simulink library "ddm"  (R2021b)
settings: Solver=VariableStepAuto  StartTime=0.0  StopTime=10.0  RelTol=1e-3
undefined symbols (not defined in the file or in its folder): ADDM_FrTMTqDev_X_Nm, ADDM_RrTMTqDev_X_Nm, ENUM_ADASACCSTA_ERROR, ENUM_ADASACCSTA_OFF, ENUM_ADASACCSTA_STANDBY, ENUM_ALLOWMOV_ALLOWREADY, ENUM_APS, ENUM_BRKSTA_ERROR, ENUM_BRKSTA_OFF, ENUM_BRKSTA_ON, ENUM_BRKSW_INVALID, ENUM_BRKSW_OFF, ENUM_BRKSW_ON, ENUM_CHGPREACTERRSTA_OBCPRE, ENUM_DCDCFAULTSTA_ANYFAULTLV1, ENUM_DCDCFAULTSTA_ANYFAULTLV2, ENUM_DRIVETRAIN_AWD, ENUM_DRIVETRAIN_FWD, ENUM_DRIVETRAIN_RWD, ENUM_EDUDRTSTA_NORMAL, ENUM_EPBSTA_APPLIED, ENUM_EPBSTA_RELEASED, ENUM_GEARACTUALPOSN_INVALID, ENUM_GEARACTUALPOSN_P, ENUM_HVBATTREADYPRE_READY, ENUM_MCUWARN_LV0, ENUM_MCUWARN_LV1, ENUM_MCUWARN_LV2, ENUM_MCUWARN_LV3, ENUM_MCUWARN_NOERROR, ENUM_OBCFAULTSTA_ANYFAULT, ENUM_PAS_R2F2, ENUM_PDFAULT_BATTPDFAIL, ENUM_PDFAULT_DCDCDISABLE, ENUM_PDFAULT_MCUDISABLE, ENUM_PDFAULT_MCUDISCHRG, ENUM_POWERSTA_OFF, ENUM_POWERSTA_ON, ENUM_POWERSTA_READY, ENUM_POWERSTA_STANDBY, ENUM_PRESSINDI_LOW, ENUM_PUFAULT_BATTUPFAIL, ENUM_PUFAULT_DCDCENABLEFAIL, ENUM_PUFAULT_PRECHRGCHKFAIL, ENUM_PUFAULT_SAFETYCHKFAIL, ENUM_PUSTATE_COMPLETED, ENUM_PWRSTASW_OFF, ENUM_PWRSTASW_OFFA, ENUM_PWRSTASW_OFFCHVCHRG, ENUM_PWRSTASW_OFFCLVCHRG, ENUM_PWRSTASW_ON, ENUM_PWRSTASW_ONHVCHRG, ENUM_PWRSTASW_READY, ENUM_PWRSTASW_STANDBY, ENUM_SHIFTCOMMAND_P, ENUM_SHIFTERERRSTA_PBUTTONFAILURE, ENUM_VEHMALFUNLV_2ND, ENUM_VEHMALFUNLV_3RD, ENUM_VEHMALFUNLV_4TH, ENUM_VEHMALFUNLV_NORMAL ... (+459)
libraries: hcu_lib x515, simulink x3
(part 5 of 25)

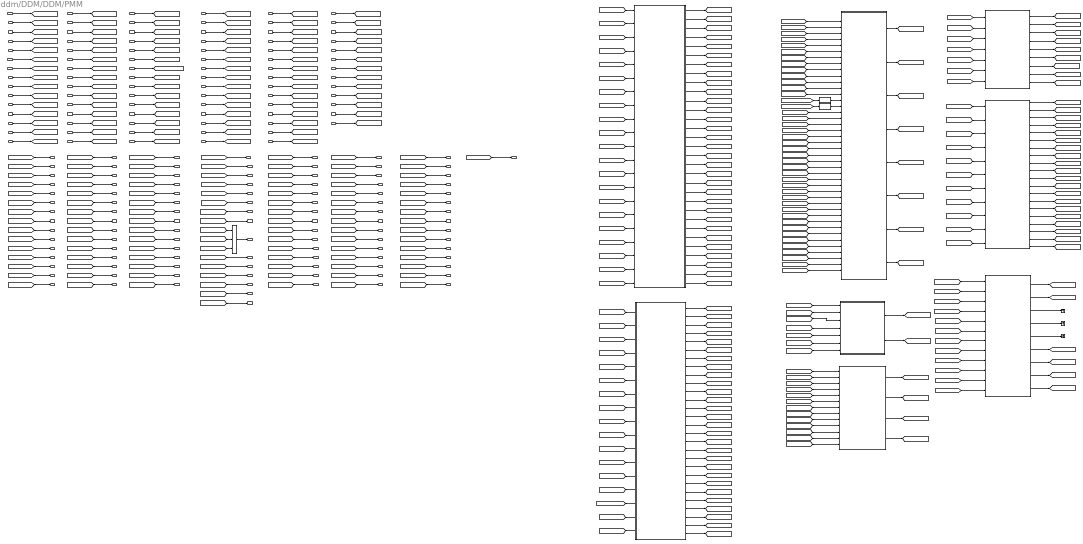
== system ddm/DDM/DDM/PMM ==
  task_time_s : Inport
  VINP_CANMsgValidABM1_flg : Inport  Port=2
  VINP_BrkPedalPosSta_enum : Inport  Port=3
  VINP_BrkPedalPos_pct : Inport  Port=4
  VINP_BrkSWSta_flg : Inport  Port=5
  VINP_CANMsgValidBMS1_flg : Inport  Port=6
  VINP_CANMsgValidBMS6_flg : Inport  Port=7
  VINP_CANMsgValidCCU1_flg : Inport  Port=8
  VINP_CANMsgValidCCU2_flg : Inport  Port=9
  VINP_BMSWarn1_flg : Inport  Port=10
  VINP_BMSWarn2_flg : Inport  Port=11
  VINP_BMSWarn3_flg : Inport  Port=12
  VINP_BMSWarn4_flg : Inport  Port=13
  VINP_BMSWarn5_flg : Inport  Port=14
  VINP_BMSWarn6_flg : Inport  Port=15
  VINP_BMSWarn7_flg : Inport  Port=16
  VINP_BMSWarn8_flg : Inport  Port=17
  VINP_DCDCFaultSta_enum : Inport  Port=18
  VINP_OBCFaultSta_enum : Inport  Port=19
  VINP_MCUWarnFNidec_enum : Inport  Port=20
  VINP_MCUWarnRNidec_enum : Inport  Port=21
  VINP_LVBattDet12V_V : Inport  Port=22
  VINP_BMSREADY_flg : Inport  Port=23
  VINP_HVBattReady4Pre_enum : Inport  Port=24
  VINP_HVBContactorSta_flg : Inport  Port=25
  VINP_DCDCReady4Pre_flg : Inport  Port=26
  VINP_DCDCEnabled_flg : Inport  Port=27
  VINP_CANMsgValidBMS5_flg : Inport  Port=28
  VINP_DrStdAErrSta_enum : Inport  Port=29
  VPMM_PowerSta_enum : Inport  Port=30
  VPMM_PwrStaSW_enum : Inport  Port=31
  VPMM_PowerUpFault_enum : Inport  Port=32
  VPMM_PowerDownFault_enum : Inport  Port=33
  VPMM_DrivetrainSelect_enum : Inport  Port=34
  VPMM_SafetyChkHLv_flg : Inport  Port=35
  VPMM_SafetyChkMLv_flg : Inport  Port=36
  VPMM_HVChrgPreActionErrSta_enum : Inport  Port=37
  VPMM_MCUReady_flg : Inport  Port=38
  VPMM_MCUReady4Pre_flg : Inport  Port=39
  VDDM_C3BMS6RCChk_flg : Inport  Port=40
  VDDM_C3BMS6CSChk_flg : Inport  Port=41
  VDDM_C3BMS1RCChk_flg : Inport  Port=42
  VDDM_C3BMS1CSChk_flg : Inport  Port=43
  VDDM_C3CCU1RCChk_flg : Inport  Port=44
  VDDM_C3CCU1CSChk_flg : Inport  Port=45
  VDDM_C3CCU2RCChk_flg : Inport  Port=46
  VDDM_C3CCU2CSChk_flg : Inport  Port=47
  VDDM_C1ABM1RCChk_flg : Inport  Port=48
  VDDM_C1ABM1CSChk_flg : Inport  Port=49
  VINP_BrakeSWGPIO_flg : Inport  Port=50
  VINP_BrakeLampSW_flg : Inport  Port=51
  VINP_DrStSW : Inport  Port=52
  VINP_FLAJARSW : Inport  Port=53
  VINP_FRAJARSW : Inport  Port=54
  VINP_RLAJARSW : Inport  Port=55
  VINP_RRAJARSW : Inport  Port=56
  VINP_HoodSW : Inport  Port=57
  VINP_TailgaSW : Inport  Port=58
  VDKC_DKCAuthSta_enum : Inport  Port=59
  VINP_AllowMovThd_OTA_enum : Inport  Port=60
  No_CAN1_BUS_OFF : Inport  Port=61
  No_CAN3_BUS_OFF : Inport  Port=62
  DTC_clear_request : Inport  Port=63
  VDDM_MCUNF1NoComCFS_flg : Inport  Port=64
  VDDM_MCUNR1NoComCFS_flg : Inport  Port=65
  VDDM_ESC5NoComCFS_flg : Inport  Port=66
  VDDM_ESC5RCErrCFS_flg : Inport  Port=67
  VDDM_ESC5CSErrCFS_flg : Inport  Port=68
  VPMM_PowerUpState_enum : Inport  Port=69
  VDDM_MCUNR1RCErrCFS_flg : Inport  Port=70
  VDDM_MCUNR1CSErrCFS_flg : Inport  Port=71
  VDDM_MCUNF1RCErrCFS_flg : Inport  Port=72
  VDDM_MCUNF1CSErrCFS_flg : Inport  Port=73
  VDDM_ESC1SigErr_flg : Inport  Port=74
  VDDM_ESC5SigErr_flg : Inport  Port=75
  VINP_ShifterFailsta_enum : Inport  Port=76
  VDDM_Shifter1NoComCFS_flg : Inport  Port=77
  VDDM_Shifter1RCErrCFS_flg : Inport  Port=78
  VDDM_Shifter1CSErrCFS_flg : Inport  Port=79
  No_CAN4_BUS_OFF : Inport  Port=80
  VINP_ZoneDrMalfunLevel_enum : Inport  Port=81
  VDDM_DrVCUNoComCFS_flg : Inport  Port=82
  ZoneFrMalfunLevel_enum : Inport  Port=83
  VDDM_FrVCUNoComCFS_flg : Inport  Port=84
  VDDM_AuxBattVolV_V : Inport  Port=85
  VPMM_MCUDCBusMaxVolt_V : Inport  Port=86
  VINP_CANMsgValidDKC1_flg : Inport  Port=87
  VINP_CANMsgValidDKC2_flg : Inport  Port=88
  Brake switch signal abnormal : Subsystem
  Comm err : Subsystem
  Data Type Conversion16 : DataTypeConversion  OutDataTypeStr=boolean
  Data Type Conversion49 : DataTypeConversion  OutDataTypeStr=boolean
  Fault level : Subsystem
  Key authentication failed : Subsystem
  LV : Subsystem
  Logical Operator5 : Logic  Operator=OR  Inputs=3  AllPortsSameDT=off  OutDataTypeStr=boolean
  SW failure : Subsystem
  System conditions of ON to READY not satisfied : Subsystem  AncestorBlock=ddm/DDM/DDM/PMM/System conditions of ON to READY not satisfied
  Terminator1 : Terminator
  Terminator10 : Terminator
  Terminator11 : Terminator
  power up and power down : Subsystem
  VDDM_C3BMS6RCDTC_raw32 : Outport
  VDDM_C3BMS6CSDTC_raw32 : Outport  Port=2
  VDDM_C3BMS6LCDTC_raw32 : Outport  Port=3
  VDDM_C3BMS1RCDTC_raw32 : Outport  Port=4
  VDDM_C3BMS1CSDTC_raw32 : Outport  Port=5
  VDDM_C3BMS1LCDTC_raw32 : Outport  Port=6
  VDDM_C3CCU1RCDTC_raw32 : Outport  Port=7
  VDDM_C3CCU1CSDTC_raw32 : Outport  Port=8
  VDDM_C3CCU1LCDTC_raw32 : Outport  Port=9
  VDDM_C3CCU2RCDTC_raw32 : Outport  Port=10
  VDDM_C3CCU2CSDTC_raw32 : Outport  Port=11
  VDDM_C3CCU2LCDTC_raw32 : Outport  Port=12
  VDDM_C1ABM1RCDTC_raw32 : Outport  Port=13
  VDDM_C1ABM1CSDTC_raw32 : Outport  Port=14
  VDDM_C1ABM1LCDTC_raw32 : Outport  Port=15
  VDDM_Lv1ErrDTC_raw32 : Outport  Port=16
  VDDM_Lv2ErrDTC_raw32 : Outport  Port=17
  VDDM_Lv3ErrDTC_raw32 : Outport  Port=18
  VDDM_Lv4ErrDTC_raw32 : Outport  Port=19
  VDDM_BrkSWErrDTC_raw32 : Outport  Port=20
  VDDM_BrkSWNoBacDTC_raw32 : Outport  Port=21
  VDDM_KeyAuthDTC_raw32 : Outport  Port=22
  VDDM_ONtoRdyDTC_raw32 : Outport  Port=23
  VDDM_HVB4PreDTC_raw32 : Outport  Port=24
  VDDM_MCU4PreDTC_raw32 : Outport  Port=25
  VDDM_DCDC4PreDTC_raw32 : Outport  Port=26
  VDDM_HVRlyCloDTC_raw32 : Outport  Port=27
  VDDM_BMSRdyDTC_raw32 : Outport  Port=28
  VDDM_DCDCEnaDTC_raw32 : Outport  Port=29
  VDDM_HiLvSaChkDTC_raw32 : Outport  Port=30
  VDDM_MidLvSaChkDTC_raw32 : Outport  Port=31
  VDDM_MCUDisDTC_raw32 : Outport  Port=32
  VDDM_DCDCDisDTC_raw32 : Outport  Port=33
  VDDM_HVRlyOpDTC_raw32 : Outport  Port=34
  VDDM_MCUActDTC_raw32 : Outport  Port=35
  VDDM_OBC4PreDTC_raw32 : Outport  Port=36
  VDDM_IniLVLoDTC_raw32 : Outport  Port=37
  VDDM_LVSupLoDTC_raw32 : Outport  Port=38
  VDDM_LVSupHiDTC_raw32 : Outport  Port=39
  VDDM_LVInErrDTC_raw32 : Outport  Port=40
  VDDM_DrStSWDTC_raw32 : Outport  Port=41
  VDDM_FLDoorSWDTC_raw32 : Outport  Port=42
  VDDM_RLDoorSWDTC_raw32 : Outport  Port=43
  VDDM_FRDoorSWDTC_raw32 : Outport  Port=44
  VDDM_RRDoorSWDTC_raw32 : Outport  Port=45
  VDDM_HoodSWDTC_raw32 : Outport  Port=46
  VDDM_TailgaSWDTC_raw32 : Outport  Port=47
  VDDM_VCUFLDoorSta_flg : Outport  Port=48
  VDDM_VCUFRDoorSta_flg : Outport  Port=49
  VDDM_VCURLDoorSta_flg : Outport  Port=50
  VDDM_VCURRDoorSta_flg : Outport  Port=51
  VDDM_VCUHoodSWSta_flg : Outport  Port=52
  VDDM_VCUTailgateSWSta_flg : Outport  Port=53
  VDDM_EDriveSysErrPMM_flg : Outport  Port=54
  VDDM_VCUBrkSWSta_enum : Outport  Port=55
  VDDM_SysAllowReadySta_flg : Outport  Port=56
  VDDM_HVRlyOpFail_flg : Outport  Port=57
  VDDM_MCUActDisFail_flg : Outport  Port=58
  VDDM_C3BMS6CSCFS_flg : Outport  Port=59
  VDDM_C3BMS6RCCFS_flg : Outport  Port=60
  VDDM_C3BMS6LCCFS_flg : Outport  Port=61
  VDDM_C3CCU2CSCFS_flg : Outport  Port=62
  VDDM_C3CCU2LCCFS_flg : Outport  Port=63
  VDDM_C3CCU2RCCFS_flg : Outport  Port=64
  VDDM_C3BMS1RCCFS_flg : Outport  Port=65
  VDDM_C3BMS1CSCFS_flg : Outport  Port=66
  VDDM_C3BMS1LCCFS_flg : Outport  Port=67
  VDDM_C3CCU1RCCFS_flg : Outport  Port=68
  VDDM_C3CCU1CSCFS_flg : Outport  Port=69
  VDDM_C3CCU1LCCFS_flg : Outport  Port=70
  VDDM_C1ABM1RCCFS_flg : Outport  Port=71
  VDDM_C1ABM1CSCFS_flg : Outport  Port=72
  VDDM_C1ABM1LCCFS_flg : Outport  Port=73
  VDDM_Lv1ErrCFS_flg : Outport  Port=74
  VDDM_Lv2ErrCFS_flg : Outport  Port=75
  VDDM_Lv3ErrCFS_flg : Outport  Port=76
  VDDM_Lv4ErrCFS_flg : Outport  Port=77
  VDDM_IniLVLoCFS_flg : Outport  Port=78
  VDDM_LVSupLoCFS_flg : Outport  Port=79
  VDDM_LVSupHiCFS_flg : Outport  Port=80
  VDDM_LVInErrCFS_flg : Outport  Port=81
  VDDM_HVB4PreCFS_flg : Outport  Port=82
  VDDM_MCU4PreCFS_flg : Outport  Port=83
  VDDM_DCDC4PreCFS_flg : Outport  Port=84
  VDDM_HVRlyCloCFS_flg : Outport  Port=85
  VDDM_BMSRdyCFS_flg : Outport  Port=86
  VDDM_DCDCEnaCFS_flg : Outport  Port=87
  VDDM_HiLvSaChkCFS_flg : Outport  Port=88
  VDDM_MidLvSaChkCFS_flg : Outport  Port=89
  VDDM_MCUDisCFS_flg : Outport  Port=90
  VDDM_DCDCDisCFS_flg : Outport  Port=91
  VDDM_HVRlyOpCFS_flg : Outport  Port=92
  VDDM_MCUActCFS_flg : Outport  Port=93
  VDDM_OBC4PreCFS_flg : Outport  Port=94
  VDDM_KeyAuthCFS_flg : Outport  Port=95
  VDDM_ONtoRdyCFS_flg : Outport  Port=96
  VDDM_DrStSWCFS_flg : Outport  Port=97
  VDDM_FLDoorSWCFS_flg : Outport  Port=98
  VDDM_RLDoorSWCFS_flg : Outport  Port=99
  VDDM_FRDoorSWCFS_flg : Outport  Port=100
  VDDM_RRDoorSWCFS_flg : Outport  Port=101
  VDDM_HoodSWCFS_flg : Outport  Port=102
  VDDM_TailgaSWCFS_flg : Outport  Port=103
  VDDM_BrkSWErrCFS_flg : Outport  Port=104
  VDDM_BrkSWNoBacCFS_flg : Outport  Port=105
  VDDM_PMMBattErr_flg : Outport  Port=106
  wires:
  [VDDM_SysAllowReadySta_flg] -> VDDM_SysAllowReadySta_flg/1
  [VDDM_VCUBrkSWSta_enum] -> VDDM_VCUBrkSWSta_enum/1
  [VDDM_C3CCU2RCCFS_flg] -> VDDM_C3CCU2RCCFS_flg/1
  [VDDM_C3CCU2LCCFS_flg] -> VDDM_C3CCU2LCCFS_flg/1
  [VDDM_C3CCU2CSCFS_flg] -> VDDM_C3CCU2CSCFS_flg/1
  [VDDM_C3BMS6LCCFS_flg] -> VDDM_C3BMS6LCCFS_flg/1
  [VDDM_C3BMS6RCCFS_flg] -> VDDM_C3BMS6RCCFS_flg/1
  [VDDM_C3BMS6CSCFS_flg] -> VDDM_C3BMS6CSCFS_flg/1
  Comm err/17(VDDM_C3BMS6CSCFS_flg) -> [VDDM_C3BMS6CSCFS_flg]
  [VPMM_PowerUpState_enum] -> power up and power down/16(VPMM_PowerUpState_enum)
  VPMM_PowerUpState_enum/1 -> [VPMM_PowerUpState_enum]
  Data Type Conversion16/1 -> Fault level/15(VDDM_C3CCU2LCCFS_flg)
  [VDDM_C3CCU2LCDTC_raw32] -> Data Type Conversion16/1
  Data Type Conversion49/1 -> Fault level/14(VDDM_C3BMS6LCCFS_flg)
  [No_CAN3_BUS_OFF] -> Fault level/22(No_CAN3_BUS_OFF)
  [DTC_clear_request] -> Fault level/21(DTC_clear_request)
  [VDDM_C3BMS6LCDTC_raw32] -> Data Type Conversion49/1
  VDDM_ESC5CSErrCFS_flg/1 -> [VDDM_ESC5CSErrCFS_flg]
  VDDM_ESC5RCErrCFS_flg/1 -> [VDDM_ESC5RCErrCFS_flg]
  VDDM_ESC5NoComCFS_flg/1 -> [VDDM_ESC5NoComCFS_flg]
  VDDM_MCUNR1NoComCFS_flg/1 -> [VDDM_MCUNR1NoComCFS_flg]
  VDDM_MCUNF1NoComCFS_flg/1 -> [VDDM_MCUNF1NoComCFS_flg]
  [VDDM_KeyAuthDTC_raw32] -> VDDM_KeyAuthDTC_raw32/1
  Brake switch signal abnormal/5(VDDM_BrkPedalPosSta_enum) -> Terminator11/1
  Brake switch signal abnormal/4(VDDM_CANBrkSW2Sta_enum) -> Terminator10/1
  System conditions of ON to READY not satisfied/4(VDDM_SysAllowReadySta_flg) -> [VDDM_SysAllowReadySta_flg]
  [VDDM_C3BMS6CSDTC_raw32] -> VDDM_C3BMS6CSDTC_raw32/1
  [VDDM_C3BMS6LCDTC_raw32] -> VDDM_C3BMS6LCDTC_raw32/1
  [VDDM_C3BMS1RCDTC_raw32] -> VDDM_C3BMS1RCDTC_raw32/1
  [VDDM_C3BMS6RCDTC_raw32] -> VDDM_C3BMS6RCDTC_raw32/1
  [VDDM_C1ABM1LCDTC_raw32] -> VDDM_C1ABM1LCDTC_raw32/1
  [VDDM_C1ABM1CSDTC_raw32] -> VDDM_C1ABM1CSDTC_raw32/1
  [VDDM_C1ABM1RCDTC_raw32] -> VDDM_C1ABM1RCDTC_raw32/1
  [VDDM_C3CCU2LCDTC_raw32] -> VDDM_C3CCU2LCDTC_raw32/1
  [VDDM_C3CCU2CSDTC_raw32] -> VDDM_C3CCU2CSDTC_raw32/1
  [VDDM_C3CCU2RCDTC_raw32] -> VDDM_C3CCU2RCDTC_raw32/1
  [VDDM_C3CCU1LCDTC_raw32] -> VDDM_C3CCU1LCDTC_raw32/1
  [VDDM_C3CCU1CSDTC_raw32] -> VDDM_C3CCU1CSDTC_raw32/1
  [VDDM_C3CCU1RCDTC_raw32] -> VDDM_C3CCU1RCDTC_raw32/1
  [VDDM_C3BMS1LCDTC_raw32] -> VDDM_C3BMS1LCDTC_raw32/1
  [VDDM_C3BMS1CSDTC_raw32] -> VDDM_C3BMS1CSDTC_raw32/1
  Comm err/15(VDDM_C1ABM1LCDTC_raw32) -> [VDDM_C1ABM1LCDTC_raw32]
  Comm err/14(VDDM_C1ABM1CSDTC_raw32) -> [VDDM_C1ABM1CSDTC_raw32]
  Comm err/13(VDDM_C1ABM1RCDTC_raw32) -> [VDDM_C1ABM1RCDTC_raw32]
  Comm err/12(VDDM_C3CCU2LCDTC_raw32) -> [VDDM_C3CCU2LCDTC_raw32]
  Comm err/11(VDDM_C3CCU2CSDTC_raw32) -> [VDDM_C3CCU2CSDTC_raw32]
  Comm err/10(VDDM_C3CCU2RCDTC_raw32) -> [VDDM_C3CCU2RCDTC_raw32]
  Comm err/9(VDDM_C3CCU1LCDTC_raw32) -> [VDDM_C3CCU1LCDTC_raw32]
  Comm err/8(VDDM_C3CCU1CSDTC_raw32) -> [VDDM_C3CCU1CSDTC_raw32]
  Comm err/7(VDDM_C3CCU1RCDTC_raw32) -> [VDDM_C3CCU1RCDTC_raw32]
  Comm err/6(VDDM_C3BMS1LCDTC_raw32) -> [VDDM_C3BMS1LCDTC_raw32]
  Comm err/5(VDDM_C3BMS1CSDTC_raw32) -> [VDDM_C3BMS1CSDTC_raw32]
  Comm err/4(VDDM_C3BMS1RCDTC_raw32) -> [VDDM_C3BMS1RCDTC_raw32]
  Comm err/3(VDDM_C3BMS6LCDTC_raw32) -> [VDDM_C3BMS6LCDTC_raw32]
  Comm err/2(VDDM_C3BMS6CSDTC_raw32) -> [VDDM_C3BMS6CSDTC_raw32]
  Comm err/1(VDDM_C3BMS6RCDTC_raw32) -> [VDDM_C3BMS6RCDTC_raw32]
  [VPMM_PwrStaSW_enum] -> Key authentication failed/3(VPMM_PwrStaSW_enum)
  [VPMM_PowerSta_enum] -> System conditions of ON to READY not satisfied/2(VPMM_PowerSta_enum)
  System conditions of ON to READY not satisfied/3(VDDM_EDriveSysErrONtoRdy_flg) -> [VDDM_EDriveSysErrONtoRdy_flg]
  [DTC_clear_request] -> Brake switch signal abnormal/12(DTC_clear_request)
  [VINP_LVBattDet12V_V] -> LV/4(VINP_LVBattDet12V_V)
  No_CAN3_BUS_OFF/1 -> [No_CAN3_BUS_OFF]
  VDDM_C3BMS1CSChk_flg/1 -> [VDDM_C3BMS1CSChk_flg]
  [VDDM_EDriveSysErrBrake_flg] -> Logical Operator5/3
  [DTC_clear_request] -> LV/6(DTC_clear_request)
  [VDDM_MCUNF1NoComCFS_flg] -> Fault level/16(VDDM_MCUNF1NoComCFS_flg)
  DTC_clear_request/1 -> [DTC_clear_request]
  [VDDM_ESC5RCErrCFS_flg] -> Brake switch signal abnormal/6(VDDM_ESC5RCErrCFS_flg)
  [VDDM_EDriveSysErrONtoRdy_flg] -> Logical Operator5/2
  [VDDM_KeyAuthCFS_flg] -> System conditions of ON to READY not satisfied/7(VDDM_KeyAuthCFS_flg)
  [VDDM_MCUNR1NoComCFS_flg] -> Fault level/17(VDDM_MCUNR1NoComCFS_flg)
  [VPMM_PowerSta_enum] -> Comm err/2(VPMM_PowerSta_enum)
  [VPMM_PowerSta_enum] -> LV/3(VPMM_PowerSta_enum)
  [DTC_clear_request] -> SW failure/4(DTC_clear_request)
  [VDDM_C3CCU1RCChk_flg] -> Comm err/10(VDDM_C3CCU1RCChk_flg)
  [DTC_clear_request] -> System conditions of ON to READY not satisfied/4(DTC_clear_request)
  [VDDM_C1ABM1RCChk_flg] -> Comm err/16(VDDM_C1ABM1RCChk_flg)
  VPMM_PowerSta_enum/1 -> [VPMM_PowerSta_enum]
  [VDDM_ESC5CSErrCFS_flg] -> Brake switch signal abnormal/7(VDDM_ESC5CSErrCFS_flg)
  [task_time_s] -> System conditions of ON to READY not satisfied/1(task_time_s)
  Logical Operator5/1 -> VDDM_EDriveSysErrPMM_flg/1
  VINP_CANMsgValidABM1_flg/1 -> [VDDM_C1ABM1LCChk_flg]
  [VINP_CANMsgValidBMS5_flg] -> LV/5(VINP_CANMsgValidBMS5_flg)
  [VDDM_C3CCU2LCChk_flg] -> Comm err/15(VDDM_C3CCU2LCChk_flg)
  [VDDM_C1ABM1CSChk_flg] -> Comm err/17(VDDM_C1ABM1CSChk_flg)
  VDDM_C1ABM1RCChk_flg/1 -> [VDDM_C1ABM1RCChk_flg]
  [No_CAN1_BUS_OFF] -> Comm err/20(No_CAN1_BUS_OFF)
  [VDDM_EDriveSysErrABMCAN_flg] -> Logical Operator5/1
  VDDM_C3BMS1RCChk_flg/1 -> [VDDM_C3BMS1RCChk_flg]
  [VDDM_C3CCU1LCChk_flg] -> Comm err/12(VDDM_C3CCU1LCChk_flg)
  VPMM_PwrStaSW_enum/1 -> [VPMM_PwrStaSW_enum]
  [VPMM_PowerSta_enum] -> Key authentication failed/2(VPMM_PowerSta_enum)
  [VPMM_PwrStaSW_enum] -> System conditions of ON to READY not satisfied/3(VPMM_PwrStaSW_enum)
  [VPMM_PwrStaSW_enum] -> Comm err/3(VPMM_PwrStaSW_enum)
  [DTC_clear_request] -> power up and power down/6(DTC_clear_request)
  [VDDM_C1ABM1LCChk_flg] -> Comm err/18(VDDM_C1ABM1LCChk_flg)
  VDDM_C3CCU2RCChk_flg/1 -> [VDDM_C3CCU2RCChk_flg]
  [task_time_s] -> power up and power down/1(task_time_s)
  [task_time_s] -> LV/1(task_time_s)
  [VDDM_C3CCU1CSChk_flg] -> Comm err/11(VDDM_C3CCU1CSChk_flg)
  [VPMM_PowerSta_enum] -> power up and power down/3(VPMM_PowerSta_enum)
  VDDM_C1ABM1CSChk_flg/1 -> [VDDM_C1ABM1CSChk_flg]
  [VDDM_C3BMS1RCChk_flg] -> Comm err/7(VDDM_C3BMS1RCChk_flg)
  VINP_CANMsgValidCCU2_flg/1 -> [VDDM_C3CCU2LCChk_flg]
  [VPMM_PwrStaSW_enum] -> LV/2(VPMM_PwrStaSW_enum)
  Brake switch signal abnormal/3(VDDM_BrakeSW_enum) -> Terminator1/1
  VINP_LVBattDet12V_V/1 -> [VINP_LVBattDet12V_V]
  [task_time_s] -> Comm err/1(task_time_s)
  Comm err/31(VDDM_EDriveSysErrABMCAN_flg) -> [VDDM_EDriveSysErrABMCAN_flg]
  [VDDM_C3CCU2CSChk_flg] -> Comm err/14(VDDM_C3CCU2CSChk_flg)
  VINP_BrakeLampSW_flg/1 -> [VINP_BrakeLampSW_flg]
  [VPMM_PowerSta_enum] -> Brake switch signal abnormal/2(VPMM_PowerSta_enum)
  VDDM_C3CCU1RCChk_flg/1 -> [VDDM_C3CCU1RCChk_flg]
  [task_time_s] -> Fault level/1(task_time_s)
  [VPMM_PowerSta_enum] -> Fault level/3(VPMM_PowerSta_enum)
  [VDDM_C3BMS6CSChk_flg] -> Comm err/5(VDDM_C3BMS6CSChk_flg)
  [VINP_BrakeLampSW_flg] -> Brake switch signal abnormal/4(VINP_BrakeLampSW_flg)
  VDDM_C3BMS6CSChk_flg/1 -> [VDDM_C3BMS6CSChk_flg]
  VINP_BrakeSWGPIO_flg/1 -> [VINP_BrakeSWGPIO_flg]
  [VPMM_PwrStaSW_enum] -> SW failure/2(VPMM_PwrStaSW_enum)
  [VDDM_C3BMS6RCChk_flg] -> Comm err/4(VDDM_C3BMS6RCChk_flg)
  [VDDM_ESC5NoComCFS_flg] -> Brake switch signal abnormal/5(VDDM_ESC5NoComCFS_flg)
  [No_CAN3_BUS_OFF] -> Comm err/19(No_CAN3_BUS_OFF)
  [task_time_s] -> SW failure/1(task_time_s)
  [VPMM_PwrStaSW_enum] -> power up and power down/2(VPMM_PwrStaSW_enum)
  [task_time_s] -> Brake switch signal abnormal/1(task_time_s)
  [DTC_clear_request] -> Comm err/21(DTC_clear_request)
  [VPMM_PowerSta_enum] -> SW failure/3(VPMM_PowerSta_enum)
  VDDM_C3BMS6RCChk_flg/1 -> [VDDM_C3BMS6RCChk_flg]
  VINP_CANMsgValidBMS6_flg/1 -> [VDDM_C3BMS6LCChk_flg]
  [DTC_clear_request] -> Key authentication failed/4(DTC_clear_request)
  [task_time_s] -> Key authentication failed/1(task_time_s)
  VDDM_C3CCU1CSChk_flg/1 -> [VDDM_C3CCU1CSChk_flg]
  VDDM_C3CCU2CSChk_flg/1 -> [VDDM_C3CCU2CSChk_flg]
  [VPMM_PwrStaSW_enum] -> Fault level/2(VPMM_PwrStaSW_enum)
  [VDDM_C3CCU2RCChk_flg] -> Comm err/13(VDDM_C3CCU2RCChk_flg)
  [VINP_BrakeSWGPIO_flg] -> Brake switch signal abnormal/3(VINP_BrakeSWGPIO_flg)
  [VDDM_C3BMS1LCChk_flg] -> Comm err/9(VDDM_C3BMS1LCChk_flg)
  task_time_s/1 -> [task_time_s]
  No_CAN1_BUS_OFF/1 -> [No_CAN1_BUS_OFF]
  [VDDM_C3BMS1CSChk_flg] -> Comm err/8(VDDM_C3BMS1CSChk_flg)
  VINP_CANMsgValidCCU1_flg/1 -> [VDDM_C3CCU1LCChk_flg]
  [VDDM_C3BMS6LCChk_flg] -> Comm err/6(VDDM_C3BMS6LCChk_flg)
  Comm err/16(VDDM_C3BMS6RCCFS_flg) -> [VDDM_C3BMS6RCCFS_flg]
  Comm err/18(VDDM_C3BMS6LCCFS_flg) -> [VDDM_C3BMS6LCCFS_flg]
  Comm err/19(VDDM_C3BMS1RCCFS_flg) -> [VDDM_C3BMS1RCCFS_flg]
  Comm err/20(VDDM_C3BMS1CSCFS_flg) -> [VDDM_C3BMS1CSCFS_flg]
  Comm err/21(VDDM_C3BMS1LCCFS_flg) -> [VDDM_C3BMS1LCCFS_flg]
  Comm err/22(VDDM_C3CCU1RCCFS_flg) -> [VDDM_C3CCU1RCCFS_flg]
  Comm err/23(VDDM_C3CCU1CSCFS_flg) -> [VDDM_C3CCU1CSCFS_flg]
  Comm err/24(VDDM_C3CCU1LCCFS_flg) -> [VDDM_C3CCU1LCCFS_flg]
  Comm err/25(VDDM_C3CCU2RCCFS_flg) -> [VDDM_C3CCU2RCCFS_flg]
  Comm err/26(VDDM_C3CCU2CSCFS_flg) -> [VDDM_C3CCU2CSCFS_flg]
  Comm err/27(VDDM_C3CCU2LCCFS_flg) -> [VDDM_C3CCU2LCCFS_flg]
  Comm err/28(VDDM_C1ABM1RCCFS_flg) -> [VDDM_C1ABM1RCCFS_flg]
  Comm err/29(VDDM_C1ABM1CSCFS_flg) -> [VDDM_C1ABM1CSCFS_flg]
  Comm err/30(VDDM_C1ABM1LCCFS_flg) -> [VDDM_C1ABM1LCCFS_flg]
  power up and power down/16(VDDM_HVB4PreCFS_flg) -> [VDDM_HVB4PreCFS_flg]
  power up and power down/17(VDDM_MCU4PreCFS_flg) -> [VDDM_MCU4PreCFS_flg]
  power up and power down/18(VDDM_DCDC4PreCFS_flg) -> [VDDM_DCDC4PreCFS_flg]
  power up and power down/19(VDDM_HVRlyCloCFS_flg) -> [VDDM_HVRlyCloCFS_flg]
  power up and power down/20(VDDM_BMSRdyCFS_flg) -> [VDDM_BMSRdyCFS_flg]
  power up and power down/21(VDDM_DCDCEnaCFS_flg) -> [VDDM_DCDCEnaCFS_flg]
  power up and power down/22(VDDM_HiLvSaChkCFS_flg) -> [VDDM_HiLvSaChkCFS_flg]
  power up and power down/23(VDDM_MidLvSaChkCFS_flg) -> [VDDM_MidLvSaChkCFS_flg]
  power up and power down/24(VDDM_MCUDisCFS_flg) -> [VDDM_MCUDisCFS_flg]
  power up and power down/25(VDDM_DCDCDisCFS_flg) -> [VDDM_DCDCDisCFS_flg]
  power up and power down/26(VDDM_HVRlyOpCFS_flg) -> [VDDM_HVRlyOpCFS_flg]
  power up and power down/27(VDDM_MCUActCFS_flg) -> [VDDM_MCUActCFS_flg]
  power up and power down/28(VDDM_OBC4PreCFS_flg) -> [VDDM_OBC4PreCFS_flg]
  Fault level/5(VDDM_Lv1ErrCFS_flg) -> [VDDM_Lv1ErrCFS_flg]
  Fault level/6(VDDM_Lv2ErrCFS_flg) -> [VDDM_Lv2ErrCFS_flg]
  Fault level/7(VDDM_Lv3ErrCFS_flg) -> [VDDM_Lv3ErrCFS_flg]
  Fault level/8(VDDM_Lv4ErrCFS_flg) -> [VDDM_Lv4ErrCFS_flg]
  LV/5(VDDM_IniLVLoCFS_flg) -> [VDDM_IniLVLoCFS_flg]
  LV/6(VDDM_LVSupLoCFS_flg) -> [VDDM_LVSupLoCFS_flg]
  LV/7(VDDM_LVSupHiCFS_flg) -> [VDDM_LVSupHiCFS_flg]
  LV/8(VDDM_LVInErrCFS_flg) -> [VDDM_LVInErrCFS_flg]
  SW failure/14(VDDM_DrStSWCFS_flg) -> [VDDM_DrStSWCFS_flg]
  SW failure/15(VDDM_FLDoorSWCFS_flg) -> [VDDM_FLDoorSWCFS_flg]
  SW failure/16(VDDM_RLDoorSWCFS_flg) -> [VDDM_RLDoorSWCFS_flg]
  SW failure/17(VDDM_FRDoorSWCFS_flg) -> [VDDM_FRDoorSWCFS_flg]
  SW failure/18(VDDM_RRDoorSWCFS_flg) -> [VDDM_RRDoorSWCFS_flg]
  SW failure/19(VDDM_HoodSWCFS_flg) -> [VDDM_HoodSWCFS_flg]
  SW failure/20(VDDM_TailgaSWCFS_flg) -> [VDDM_TailgaSWCFS_flg]
  [VDDM_C3CCU2RCCFS_flg] -> Fault level/23(VDDM_C3CCU2RCCFS_flg)
  [VDDM_C3CCU2CSCFS_flg] -> Fault level/24(VDDM_C3CCU2CSCFS_flg)
  [VDDM_MCUNR1RCErrCFS_flg] -> Fault level/25(VDDM_MCUNR1RCErrCFS_flg)
  [VDDM_MCUNR1CSErrCFS_flg] -> Fault level/26(VDDM_MCUNR1CSErrCFS_flg)
  [VDDM_MCUNF1RCErrCFS_flg] -> Fault level/27(VDDM_MCUNF1RCErrCFS_flg)
  [VDDM_MCUNF1CSErrCFS_flg] -> Fault level/28(VDDM_MCUNF1CSErrCFS_flg)
  [VDDM_C3BMS6RCCFS_flg] -> Fault level/29(VDDM_C3BMS6RCCFS_flg)
  [VDDM_C3BMS6CSCFS_flg] -> Fault level/30(VDDM_C3BMS6CSCFS_flg)
  [VDDM_ESC1SigErr_flg] -> Fault level/32(VDDM_ESC1SigErr_flg)
  [VDDM_ESC5SigErr_flg] -> Fault level/33(VDDM_ESC5SigErr_flg)
  [No_CAN1_BUS_OFF] -> Fault level/31(No_CAN1_BUS_OFF)
  [ZoneFrMalfunLevel_enum] -> Fault level/34(ZoneFrMalfunLevel_enum)
  [VDDM_FrVCUNoComCFS_flg] -> Fault level/35(VDDM_FrVCUNoComCFS_flg)
  [VINP_ShifterFailsta_enum] -> Fault level/36(VINP_ShifterFailsta_enum)
  [VDDM_Shifter1NoComCFS_flg] -> Fault level/37(VDDM_Shifter1NoComCFS_flg)
  [VDDM_Shifter1RCErrCFS_flg] -> Fault level/38(VDDM_Shifter1RCErrCFS_flg)
  [VDDM_Shifter1CSErrCFS_flg] -> Fault level/39(VDDM_Shifter1CSErrCFS_flg)
  [VINP_ZoneDrMalfunLevel_enum] -> Fault level/40(VINP_ZoneDrMalfunLevel_enum)
  [No_CAN4_BUS_OFF] -> Fault level/41(No_CAN4_BUS_OFF)
  [VDDM_DrVCUNoComCFS_flg] -> Fault level/42(VDDM_DrVCUNoComCFS_flg)
  Brake switch signal abnormal/8(VDDM_VCUBrkSWSta_enum) -> [VDDM_VCUBrkSWSta_enum]
  Brake switch signal abnormal/9(VDDM_EDriveSysErrBrake_flg) -> [VDDM_EDriveSysErrBrake_flg]
  Brake switch signal abnormal/6(VDDM_BrkSWErrCFS_flg) -> [VDDM_BrkSWErrCFS_flg]
  Brake switch signal abnormal/7(VDDM_BrkSWNoBacCFS_flg) -> [VDDM_BrkSWNoBacCFS_flg]
  Key authentication failed/1(VDDM_KeyAuthDTC_raw32) -> [VDDM_KeyAuthDTC_raw32]
  Key authentication failed/2(VDDM_KeyAuthCFS_flg) -> [VDDM_KeyAuthCFS_flg]
  [VDDM_FLDoorSWCFS_flg] -> System conditions of ON to READY not satisfied/8(VDDM_FLDoorSWCFS_flg)
  [VDDM_RLDoorSWCFS_flg] -> System conditions of ON to READY not satisfied/9(VDDM_RLDoorSWCFS_flg)
  [VDDM_RRDoorSWCFS_flg] -> System conditions of ON to READY not satisfied/11(VDDM_RRDoorSWCFS_flg)
  [VDDM_FRDoorSWCFS_flg] -> System conditions of ON to READY not satisfied/10(VDDM_FRDoorSWCFS_flg)
  [VDDM_HoodSWCFS_flg] -> System conditions of ON to READY not satisfied/12(VDDM_HoodSWCFS_flg)
  [VDDM_TailgaSWCFS_flg] -> System conditions of ON to READY not satisfied/13(VDDM_TailgaSWCFS_flg)
  System conditions of ON to READY not satisfied/2(VDDM_ONtoRdyCFS_flg) -> [VDDM_ONtoRdyCFS_flg]
  [VDDM_C3BMS1RCCFS_flg] -> VDDM_C3BMS1RCCFS_flg/1
  [VDDM_C3BMS1CSCFS_flg] -> VDDM_C3BMS1CSCFS_flg/1
  [VDDM_C3BMS1LCCFS_flg] -> VDDM_C3BMS1LCCFS_flg/1
  [VDDM_C3CCU1RCCFS_flg] -> VDDM_C3CCU1RCCFS_flg/1
  [VDDM_C3CCU1CSCFS_flg] -> VDDM_C3CCU1CSCFS_flg/1
  [VDDM_C3CCU1LCCFS_flg] -> VDDM_C3CCU1LCCFS_flg/1
  [VDDM_C1ABM1RCCFS_flg] -> VDDM_C1ABM1RCCFS_flg/1
  [VDDM_C1ABM1CSCFS_flg] -> VDDM_C1ABM1CSCFS_flg/1
  [VDDM_C1ABM1LCCFS_flg] -> VDDM_C1ABM1LCCFS_flg/1
  [VDDM_Lv1ErrCFS_flg] -> VDDM_Lv1ErrCFS_flg/1
  [VDDM_Lv2ErrCFS_flg] -> VDDM_Lv2ErrCFS_flg/1
  [VDDM_Lv3ErrCFS_flg] -> VDDM_Lv3ErrCFS_flg/1
  [VDDM_Lv4ErrCFS_flg] -> VDDM_Lv4ErrCFS_flg/1
  [VDDM_IniLVLoCFS_flg] -> VDDM_IniLVLoCFS_flg/1
  [VDDM_LVSupLoCFS_flg] -> VDDM_LVSupLoCFS_flg/1
  [VDDM_LVSupHiCFS_flg] -> VDDM_LVSupHiCFS_flg/1
  [VDDM_LVInErrCFS_flg] -> VDDM_LVInErrCFS_flg/1
  [VDDM_HVB4PreCFS_flg] -> VDDM_HVB4PreCFS_flg/1
  [VDDM_MCU4PreCFS_flg] -> VDDM_MCU4PreCFS_flg/1
  [VDDM_DCDC4PreCFS_flg] -> VDDM_DCDC4PreCFS_flg/1
  [VDDM_HVRlyCloCFS_flg] -> VDDM_HVRlyCloCFS_flg/1
  [VDDM_BMSRdyCFS_flg] -> VDDM_BMSRdyCFS_flg/1
  [VDDM_DCDCEnaCFS_flg] -> VDDM_DCDCEnaCFS_flg/1
  [VDDM_HiLvSaChkCFS_flg] -> VDDM_HiLvSaChkCFS_flg/1
  [VDDM_MidLvSaChkCFS_flg] -> VDDM_MidLvSaChkCFS_flg/1
  [VDDM_MCUDisCFS_flg] -> VDDM_MCUDisCFS_flg/1
  [VDDM_DCDCDisCFS_flg] -> VDDM_DCDCDisCFS_flg/1
  [VDDM_HVRlyOpCFS_flg] -> VDDM_HVRlyOpCFS_flg/1
  [VDDM_MCUActCFS_flg] -> VDDM_MCUActCFS_flg/1
  [VDDM_OBC4PreCFS_flg] -> VDDM_OBC4PreCFS_flg/1
  [VDDM_KeyAuthCFS_flg] -> VDDM_KeyAuthCFS_flg/1
  [VDDM_ONtoRdyCFS_flg] -> VDDM_ONtoRdyCFS_flg/1
  [VDDM_DrStSWCFS_flg] -> VDDM_DrStSWCFS_flg/1
  [VDDM_FLDoorSWCFS_flg] -> VDDM_FLDoorSWCFS_flg/1
  [VDDM_RLDoorSWCFS_flg] -> VDDM_RLDoorSWCFS_flg/1
  [VDDM_FRDoorSWCFS_flg] -> VDDM_FRDoorSWCFS_flg/1
  [VDDM_RRDoorSWCFS_flg] -> VDDM_RRDoorSWCFS_flg/1
  [VDDM_TailgaSWCFS_flg] -> VDDM_TailgaSWCFS_flg/1
  [VDDM_HoodSWCFS_flg] -> VDDM_HoodSWCFS_flg/1
  [VDDM_BrkSWErrCFS_flg] -> VDDM_BrkSWErrCFS_flg/1
  [VDDM_BrkSWNoBacCFS_flg] -> VDDM_BrkSWNoBacCFS_flg/1
  VDDM_MCUNF1CSErrCFS_flg/1 -> [VDDM_MCUNF1CSErrCFS_flg]
  VDDM_Shifter1NoComCFS_flg/1 -> [VDDM_Shifter1NoComCFS_flg]
  VINP_ShifterFailsta_enum/1 -> [VINP_ShifterFailsta_enum]
  ZoneFrMalfunLevel_enum/1 -> [ZoneFrMalfunLevel_enum]
  No_CAN4_BUS_OFF/1 -> [No_CAN4_BUS_OFF]
  VDDM_FrVCUNoComCFS_flg/1 -> [VDDM_FrVCUNoComCFS_flg]
  VINP_ZoneDrMalfunLevel_enum/1 -> [VINP_ZoneDrMalfunLevel_enum]
  VDDM_ESC5SigErr_flg/1 -> [VDDM_ESC5SigErr_flg]
  VDDM_MCUNR1CSErrCFS_flg/1 -> [VDDM_MCUNR1CSErrCFS_flg]
  VDDM_Shifter1RCErrCFS_flg/1 -> [VDDM_Shifter1RCErrCFS_flg]
  VDDM_MCUNR1RCErrCFS_flg/1 -> [VDDM_MCUNR1RCErrCFS_flg]
  VDDM_Shifter1CSErrCFS_flg/1 -> [VDDM_Shifter1CSErrCFS_flg]
  VDDM_ESC1SigErr_flg/1 -> [VDDM_ESC1SigErr_flg]
  VDDM_AuxBattVolV_V/1 -> [VDDM_AuxBattVolV_V]
  VDDM_MCUNF1RCErrCFS_flg/1 -> [VDDM_MCUNF1RCErrCFS_flg]
  VDDM_DrVCUNoComCFS_flg/1 -> [VDDM_DrVCUNoComCFS_flg]
  [VPMM_MCUDCBusMaxVolt_V] -> power up and power down/17(VPMM_MCUDCBusMaxVolt_V)
  VPMM_MCUDCBusMaxVolt_V/1 -> [VPMM_MCUDCBusMaxVolt_V]
  VINP_CANMsgValidBMS5_flg/1 -> [VINP_CANMsgValidBMS5_flg]
  [VDDM_AuxBattVolV_V] -> LV/7(VDDM_AuxBattVolV_V)
  VPMM_PowerUpFault_enum/1 -> [VPMM_PowerUpFault_enum]
  [VPMM_PowerUpFault_enum] -> power up and power down/4(VPMM_PowerUpFault_enum)
  VPMM_PowerDownFault_enum/1 -> [VPMM_PowerDownFault_enum]
  [VPMM_PowerDownFault_enum] -> power up and power down/5(VPMM_PowerDownFault_enum)
  VINP_HVBattReady4Pre_enum/1 -> [VINP_HVBattReady4Pre_enum]
  [VINP_HVBattReady4Pre_enum] -> power up and power down/7(VINP_HVBattReady4Pre_enum)
  VPMM_MCUReady4Pre_flg/1 -> [VPMM_MCUReady4Pre_flg]
  [VPMM_MCUReady4Pre_flg] -> power up and power down/8(VPMM_MCUReady4Pre_flg)
  VINP_DCDCReady4Pre_flg/1 -> [VINP_DCDCReady4Pre_flg]
  [VINP_DCDCReady4Pre_flg] -> power up and power down/9(VINP_DCDCReady4Pre_flg)
  VINP_HVBContactorSta_flg/1 -> [VINP_HVBContactorSta_flg]
  [VINP_HVBContactorSta_flg] -> power up and power down/10(VINP_HVBContactorSta_flg)
  VINP_BMSREADY_flg/1 -> [VINP_BMSREADY_flg]
  [VINP_BMSREADY_flg] -> power up and power down/11(VINP_BMSREADY_flg)
  VINP_DCDCEnabled_flg/1 -> [VINP_DCDCEnabled_flg]
  [VINP_DCDCEnabled_flg] -> power up and power down/12(VINP_DCDCEnabled_flg)
  VPMM_SafetyChkHLv_flg/1 -> [VPMM_SafetyChkHLv_flg]
  VPMM_SafetyChkMLv_flg/1 -> [VPMM_SafetyChkMLv_flg]
  [VPMM_SafetyChkHLv_flg] -> power up and power down/13(VPMM_SafetyChkHLv_flg)
  [VPMM_SafetyChkMLv_flg] -> power up and power down/14(VPMM_SafetyChkMLv_flg)
  VPMM_HVChrgPreActionErrSta_enum/1 -> [VPMM_HVChrgPreActionErrSta_enum]
  [VPMM_HVChrgPreActionErrSta_enum] -> power up and power down/15(VPMM_HVChrgPreActionErrSta_enum)
  VPMM_DrivetrainSelect_enum/1 -> [VPMM_DrivetrainSelect_enum]
  VINP_DCDCFaultSta_enum/1 -> [VINP_DCDCFaultSta_enum]
  VINP_BMSWarn1_flg/1 -> [VINP_BMSWarn1_flg]
  VINP_BMSWarn2_flg/1 -> [VINP_BMSWarn2_flg]
  VINP_BMSWarn3_flg/1 -> [VINP_BMSWarn3_flg]
  VINP_BMSWarn4_flg/1 -> [VINP_BMSWarn4_flg]
  VINP_BMSWarn5_flg/1 -> [VINP_BMSWarn5_flg]
  VINP_BMSWarn6_flg/1 -> [VINP_BMSWarn6_flg]
  VINP_BMSWarn7_flg/1 -> [VINP_BMSWarn7_flg]
  VINP_BMSWarn8_flg/1 -> [VINP_BMSWarn8_flg]
  [VINP_BMSWarn1_flg] -> Fault level/4(VINP_BMSWarn1_flg)
  [VPMM_DrivetrainSelect_enum] -> Fault level/13(VPMM_DrivetrainSelect_enum)
  [VINP_DCDCFaultSta_enum] -> Fault level/12(VINP_DCDCFaultSta_enum)
  [VINP_BMSWarn8_flg] -> Fault level/11(VINP_BMSWarn8_flg)
  [VINP_BMSWarn7_flg] -> Fault level/10(VINP_BMSWarn7_flg)
  [VINP_BMSWarn6_flg] -> Fault level/9(VINP_BMSWarn6_flg)
  [VINP_BMSWarn4_flg] -> Fault level/7(VINP_BMSWarn4_flg)
  [VINP_BMSWarn5_flg] -> Fault level/8(VINP_BMSWarn5_flg)
  [VINP_BMSWarn3_flg] -> Fault level/6(VINP_BMSWarn3_flg)
  [VINP_BMSWarn2_flg] -> Fault level/5(VINP_BMSWarn2_flg)
  [VINP_BrkPedalPosSta_enum] -> Brake switch signal abnormal/10(VINP_BrkPedalPosSta_enum)
  [VINP_BrkPedalPos_pct] -> Brake switch signal abnormal/11(VINP_BrkPedalPos_pct)
  [VINP_BrkSWSta_flg] -> Brake switch signal abnormal/9(VINP_BrkSWSta_flg)
  VINP_BrkPedalPosSta_enum/1 -> [VINP_BrkPedalPosSta_enum]
  VINP_BrkPedalPos_pct/1 -> [VINP_BrkPedalPos_pct]
  VINP_BrkSWSta_flg/1 -> [VINP_BrkSWSta_flg]
  [VINP_OBCFaultSta_enum] -> Fault level/20(VINP_OBCFaultSta_enum)
  [VINP_MCUWarnRNidec_enum] -> Fault level/19(VINP_MCUWarnRNidec_enum)
  [VINP_MCUWarnFNidec_enum] -> Fault level/18(VINP_MCUWarnFNidec_enum)
  VINP_MCUWarnFNidec_enum/1 -> [VINP_MCUWarnFNidec_enum]
  VINP_OBCFaultSta_enum/1 -> [VINP_OBCFaultSta_enum]
  VINP_MCUWarnRNidec_enum/1 -> [VINP_MCUWarnRNidec_enum]
  [VINP_DrStdAErrSta_enum] -> Brake switch signal abnormal/8(VINP_DrStdAErrSta_enum)
  VINP_DrStdAErrSta_enum/1 -> [VINP_DrStdAErrSta_enum]
  [VPMM_MCUReady_flg] -> System conditions of ON to READY not satisfied/5(VPMM_MCUReady_flg)
  VPMM_MCUReady_flg/1 -> [VPMM_MCUReady_flg]
  [VINP_DrStSW] -> SW failure/5(VINP_DrStSW)
  [VINP_FLAJARSW] -> SW failure/6(VINP_FLAJARSW)
  [VINP_FRAJARSW] -> SW failure/7(VINP_FRAJARSW)
  [VINP_RLAJARSW] -> SW failure/8(VINP_RLAJARSW)
  [VINP_RRAJARSW] -> SW failure/9(VINP_RRAJARSW)
  [VINP_HoodSW] -> SW failure/10(VINP_HoodSW)
  [VINP_TailgaSW] -> SW failure/11(VINP_TailgaSW)
  VINP_DrStSW/1 -> [VINP_DrStSW]
  VINP_FLAJARSW/1 -> [VINP_FLAJARSW]
  VINP_FRAJARSW/1 -> [VINP_FRAJARSW]
  VINP_RLAJARSW/1 -> [VINP_RLAJARSW]
  VINP_RRAJARSW/1 -> [VINP_RRAJARSW]
  VINP_HoodSW/1 -> [VINP_HoodSW]
  VINP_TailgaSW/1 -> [VINP_TailgaSW]
  [VDKC_DKCAuthSta_enum] -> Key authentication failed/5(VDKC_DKCAuthSta_enum)
  VDKC_DKCAuthSta_enum/1 -> [VDKC_DKCAuthSta_enum]
  [VINP_AllowMovThd_OTA_enum] -> System conditions of ON to READY not satisfied/6(VINP_AllowMovThd_OTA_enum)
  VINP_AllowMovThd_OTA_enum/1 -> [VINP_AllowMovThd_OTA_enum]
  Fault level/1(VDDM_Lv1ErrDTC_raw32) -> [VDDM_Lv1ErrDTC_raw32]
  Fault level/2(VDDM_Lv2ErrDTC_raw32) -> [VDDM_Lv2ErrDTC_raw32]
  Fault level/3(VDDM_Lv3ErrDTC_raw32) -> [VDDM_Lv3ErrDTC_raw32]
  Fault level/4(VDDM_Lv4ErrDTC_raw32) -> [VDDM_Lv4ErrDTC_raw32]
  [VDDM_Lv1ErrDTC_raw32] -> VDDM_Lv1ErrDTC_raw32/1
  [VDDM_Lv2ErrDTC_raw32] -> VDDM_Lv2ErrDTC_raw32/1
  [VDDM_Lv3ErrDTC_raw32] -> VDDM_Lv3ErrDTC_raw32/1
  [VDDM_Lv4ErrDTC_raw32] -> VDDM_Lv4ErrDTC_raw32/1
  Brake switch signal abnormal/2(VDDM_BrkSWNoBacDTC_raw32) -> [VDDM_BrkSWNoBacDTC_raw32]
  Brake switch signal abnormal/1(VDDM_BrkSWErrDTC_raw32) -> [VDDM_BrkSWErrDTC_raw32]
  [VDDM_BrkSWErrDTC_raw32] -> VDDM_BrkSWErrDTC_raw32/1
  [VDDM_BrkSWNoBacDTC_raw32] -> VDDM_BrkSWNoBacDTC_raw32/1
  System conditions of ON to READY not satisfied/1(VDDM_ONtoRdyDTC_raw32) -> [VDDM_ONtoRdyDTC_raw32]
  [VDDM_ONtoRdyDTC_raw32] -> VDDM_ONtoRdyDTC_raw32/1
  [VDDM_HVB4PreDTC_raw32] -> VDDM_HVB4PreDTC_raw32/1
  [VDDM_MCU4PreDTC_raw32] -> VDDM_MCU4PreDTC_raw32/1
  [VDDM_HVRlyCloDTC_raw32] -> VDDM_HVRlyCloDTC_raw32/1
  [VDDM_DCDC4PreDTC_raw32] -> VDDM_DCDC4PreDTC_raw32/1
  [VDDM_BMSRdyDTC_raw32] -> VDDM_BMSRdyDTC_raw32/1
  [VDDM_DCDCEnaDTC_raw32] -> VDDM_DCDCEnaDTC_raw32/1
  [VDDM_MidLvSaChkDTC_raw32] -> VDDM_MidLvSaChkDTC_raw32/1
  [VDDM_MCUDisDTC_raw32] -> VDDM_MCUDisDTC_raw32/1
  [VDDM_DCDCDisDTC_raw32] -> VDDM_DCDCDisDTC_raw32/1
  [VDDM_HVRlyOpDTC_raw32] -> VDDM_HVRlyOpDTC_raw32/1
  [VDDM_MCUActDTC_raw32] -> VDDM_MCUActDTC_raw32/1
  [VDDM_OBC4PreDTC_raw32] -> VDDM_OBC4PreDTC_raw32/1
  [VDDM_IniLVLoDTC_raw32] -> VDDM_IniLVLoDTC_raw32/1
  [VDDM_LVSupLoDTC_raw32] -> VDDM_LVSupLoDTC_raw32/1
  [VDDM_LVInErrDTC_raw32] -> VDDM_LVInErrDTC_raw32/1
  [VDDM_LVSupHiDTC_raw32] -> VDDM_LVSupHiDTC_raw32/1
  LV/4(VDDM_LVInErrDTC_raw32) -> [VDDM_LVInErrDTC_raw32]
  LV/3(VDDM_LVSupHiDTC_raw32) -> [VDDM_LVSupHiDTC_raw32]
  LV/2(VDDM_LVSupLoDTC_raw32) -> [VDDM_LVSupLoDTC_raw32]
  LV/1(VDDM_IniLVLoDTC_raw32) -> [VDDM_IniLVLoDTC_raw32]
  power up and power down/1(VDDM_HVB4PreDTC_raw32) -> [VDDM_HVB4PreDTC_raw32]
  power up and power down/2(VDDM_MCU4PreDTC_raw32) -> [VDDM_MCU4PreDTC_raw32]
  power up and power down/3(VDDM_DCDC4PreDTC_raw32) -> [VDDM_DCDC4PreDTC_raw32]
  power up and power down/4(VDDM_HVRlyCloDTC_raw32) -> [VDDM_HVRlyCloDTC_raw32]
  power up and power down/5(VDDM_BMSRdyDTC_raw32) -> [VDDM_BMSRdyDTC_raw32]
  power up and power down/6(VDDM_DCDCEnaDTC_raw32) -> [VDDM_DCDCEnaDTC_raw32]
  power up and power down/7(VDDM_HiLvSaChkDTC_raw32) -> [VDDM_HiLvSaChkDTC_raw32]
  power up and power down/8(VDDM_MidLvSaChkDTC_raw32) -> [VDDM_MidLvSaChkDTC_raw32]
  power up and power down/9(VDDM_MCUDisDTC_raw32) -> [VDDM_MCUDisDTC_raw32]
  power up and power down/10(VDDM_DCDCDisDTC_raw32) -> [VDDM_DCDCDisDTC_raw32]
  power up and power down/11(VDDM_HVRlyOpDTC_raw32) -> [VDDM_HVRlyOpDTC_raw32]
  power up and power down/12(VDDM_MCUActDTC_raw32) -> [VDDM_MCUActDTC_raw32]
  power up and power down/13(VDDM_OBC4PreDTC_raw32) -> [VDDM_OBC4PreDTC_raw32]
  power up and power down/14(VDDM_HVRlyOpFail_flg) -> [VDDM_HVRlyOpFail_flg]
  power up and power down/15(VDDM_MCUActDisFail_flg) -> [VDDM_MCUActDisFail_flg]
  [VDDM_HiLvSaChkDTC_raw32] -> VDDM_HiLvSaChkDTC_raw32/1
  [VDDM_DrStSWDTC_raw32] -> VDDM_DrStSWDTC_raw32/1
  [VDDM_FLDoorSWDTC_raw32] -> VDDM_FLDoorSWDTC_raw32/1
  [VDDM_RLDoorSWDTC_raw32] -> VDDM_RLDoorSWDTC_raw32/1
  [VDDM_FRDoorSWDTC_raw32] -> VDDM_FRDoorSWDTC_raw32/1
  [VDDM_RRDoorSWDTC_raw32] -> VDDM_RRDoorSWDTC_raw32/1
  [VDDM_HoodSWDTC_raw32] -> VDDM_HoodSWDTC_raw32/1
  [VDDM_TailgaSWDTC_raw32] -> VDDM_TailgaSWDTC_raw32/1
  [VDDM_VCUFLDoorSta_flg] -> VDDM_VCUFLDoorSta_flg/1
  [VDDM_VCUFRDoorSta_flg] -> VDDM_VCUFRDoorSta_flg/1
  [VDDM_VCURLDoorSta_flg] -> VDDM_VCURLDoorSta_flg/1
  [VDDM_VCURRDoorSta_flg] -> VDDM_VCURRDoorSta_flg/1
  [VDDM_VCUHoodSWSta_flg] -> VDDM_VCUHoodSWSta_flg/1
  [VDDM_VCUTailgateSWSta_flg] -> VDDM_VCUTailgateSWSta_flg/1
  [VDDM_HVRlyOpFail_flg] -> VDDM_HVRlyOpFail_flg/1
  [VDDM_MCUActDisFail_flg] -> VDDM_MCUActDisFail_flg/1
  SW failure/1(VDDM_DrStSWDTC_raw32) -> [VDDM_DrStSWDTC_raw32]
  SW failure/2(VDDM_FLDoorSWDTC_raw32) -> [VDDM_FLDoorSWDTC_raw32]
  SW failure/3(VDDM_RLDoorSWDTC_raw32) -> [VDDM_RLDoorSWDTC_raw32]
  SW failure/4(VDDM_FRDoorSWDTC_raw32) -> [VDDM_FRDoorSWDTC_raw32]
  SW failure/5(VDDM_RRDoorSWDTC_raw32) -> [VDDM_RRDoorSWDTC_raw32]
  SW failure/6(VDDM_HoodSWDTC_raw32) -> [VDDM_HoodSWDTC_raw32]
  SW failure/7(VDDM_TailgaSWDTC_raw32) -> [VDDM_TailgaSWDTC_raw32]
  SW failure/8(VDDM_VCUFLDoorSta_flg) -> [VDDM_VCUFLDoorSta_flg]
  SW failure/9(VDDM_VCUFRDoorSta_flg) -> [VDDM_VCUFRDoorSta_flg]
  SW failure/10(VDDM_VCURLDoorSta_flg) -> [VDDM_VCURLDoorSta_flg]
  SW failure/11(VDDM_VCURRDoorSta_flg) -> [VDDM_VCURRDoorSta_flg]
  SW failure/12(VDDM_VCUHoodSWSta_flg) -> [VDDM_VCUHoodSWSta_flg]
  SW failure/13(VDDM_VCUTailgateSWSta_flg) -> [VDDM_VCUTailgateSWSta_flg]
  [VINP_CANMsgValidDKC2_flg] -> Key authentication failed/6(VINP_CANMsgValidDKC2_flg)
  [VINP_CANMsgValidDKC1_flg] -> Key authentication failed/7(VINP_CANMsgValidDKC1_flg)
  VINP_CANMsgValidDKC1_flg/1 -> [VINP_CANMsgValidDKC1_flg]
  VINP_CANMsgValidDKC2_flg/1 -> [VINP_CANMsgValidDKC2_flg]
  LV/9(VDDM_PMMBattErr_flg) -> [VDDM_PMMBattErr_flg]
  [VDDM_PMMBattErr_flg] -> VDDM_PMMBattErr_flg/1
  VINP_CANMsgValidBMS1_flg/1 -> [VDDM_C3BMS1LCChk_flg]

== system ddm/DDM/DDM/TPM ==
  note: SensorFail
  note: WheelTmpHigh
  note: PressureLow
  note: Batwarn
  task_time_s : Inport
  VPMM_PowerSta_enum : Inport  Port=2
  DTC_clear_request : Inport  Port=3
  VTPM_LFBatwarn_flg : Inport  Port=4
  VTPM_RFBatwarn_flg : Inport  Port=5
  VTPM_LRBatwarn_flg : Inport  Port=6
  VTPM_RRBatwarn_flg : Inport  Port=7
  VTPM_LFPressIndi_enum : Inport  Port=8
  VTPM_RFPressIndi_enum : Inport  Port=9
  VTPM_LRPressIndi_enum : Inport  Port=10
  VTPM_RRPressIndi_enum : Inport  Port=11
  VTPM_LFWheelTmpIndi_flg : Inport  Port=12
  VTPM_RFWheelTmpIndi_flg : Inport  Port=13
  VTPM_LRWheelTmpIndi_flg : Inport  Port=14
  VTPM_RRWheelTmpIndi_flg : Inport  Port=15
  VTPM_LFSensorFail_flg : Inport  Port=16
  VTPM_RFSensorFail_flg : Inport  Port=17
  VTPM_LRSensorFail_flg : Inport  Port=18
  VTPM_RRSensorFail_flg : Inport  Port=19
  LFBatwarn : Subsystem
  LFPressureLow : Subsystem
  LFSensorfail : Subsystem
  LFWheelTmpHigh : Subsystem
  LRBatwarn : Subsystem
  LRPressureLow : Subsystem
  LRSensorfail : Subsystem
  LRWheelTmpHigh : Subsystem
  RFBatwarn : Subsystem
  RFPressureLow : Subsystem
  RFSensorfail : Subsystem
  RFWheelTmpHigh : Subsystem
  RRBatwarn : Subsystem
  RRPressureLow : Subsystem
  RRSensorfail : Subsystem
  RRWheelTmpHigh : Subsystem
  VDDM_LFBatwarnDTC_raw32 : Outport
  VDDM_RFBatwarnDTC_raw32 : Outport  Port=2
  VDDM_LRBatwarnDTC_raw32 : Outport  Port=3
  VDDM_RRBatwarnDTC_raw32 : Outport  Port=4
  VDDM_LFPressIndiDTC_raw32 : Outport  Port=5
  VDDM_RFPressIndiDTC_raw32 : Outport  Port=6
  VDDM_LRPressIndiDTC_raw32 : Outport  Port=7
  VDDM_RRPressIndiDTC_raw32 : Outport  Port=8
  VDDM_LFWheelTmpHighDTC_raw32 : Outport  Port=9
  VDDM_RFWheelTmpHighDTC_raw32 : Outport  Port=10
  VDDM_LRWheelTmpHighDTC_raw32 : Outport  Port=11
  VDDM_RRWheelTmpHighDTC_raw32 : Outport  Port=12
  VDDM_LFSensorFailDTC_raw32 : Outport  Port=13
  VDDM_RFSensorFailDTC_raw32 : Outport  Port=14
  VDDM_LRSensorFailDTC_raw32 : Outport  Port=15
  VDDM_RRSensorFailDTC_raw32 : Outport  Port=16
  wires:
  VPMM_PowerSta_enum/1 -> [VPMM_PowerSta_enum]
  DTC_clear_request/1 -> [DTC_clear_request]
  task_time_s/1 -> [task_time_s]
  [VPMM_PowerSta_enum] -> LFBatwarn/2(VPMM_PowerSta_enum)
  [task_time_s] -> LFBatwarn/1(task_time_s)
  [DTC_clear_request] -> LFBatwarn/3(DTC_clear_request)
  VTPM_LFBatwarn_flg/1 -> LFBatwarn/4(VTPM_LFBatwarn_flg)
  LFBatwarn/1(VDDM_LFBatwarnDTC_raw32) -> VDDM_LFBatwarnDTC_raw32/1
  [task_time_s] -> RFBatwarn/1(task_time_s)
  [VPMM_PowerSta_enum] -> RFBatwarn/2(VPMM_PowerSta_enum)
  [DTC_clear_request] -> RFBatwarn/3(DTC_clear_request)
  VTPM_RFBatwarn_flg/1 -> RFBatwarn/4(VTPM_RFBatwarn_flg)
  RFBatwarn/1(VDDM_RFBatwarnDTC_raw32) -> VDDM_RFBatwarnDTC_raw32/1
  [task_time_s] -> LRBatwarn/1(task_time_s)
  [VPMM_PowerSta_enum] -> LRBatwarn/2(VPMM_PowerSta_enum)
  [DTC_clear_request] -> LRBatwarn/3(DTC_clear_request)
  VTPM_LRBatwarn_flg/1 -> LRBatwarn/4(VTPM_LRBatwarn_flg)
  LRBatwarn/1(VDDM_LRBatwarnDTC_raw32) -> VDDM_LRBatwarnDTC_raw32/1
  RRBatwarn/1(VDDM_RRBatwarnDTC_raw32) -> VDDM_RRBatwarnDTC_raw32/1
  [task_time_s] -> RRBatwarn/1(task_time_s)
  [VPMM_PowerSta_enum] -> RRBatwarn/2(VPMM_PowerSta_enum)
  [DTC_clear_request] -> RRBatwarn/3(DTC_clear_request)
  VTPM_RRBatwarn_flg/1 -> RRBatwarn/4(VTPM_RRBatwarn_flg)
  [task_time_s] -> LFPressureLow/1(task_time_s)
  [VPMM_PowerSta_enum] -> LFPressureLow/2(VPMM_PowerSta_enum)
  [DTC_clear_request] -> LFPressureLow/3(DTC_clear_request)
  [task_time_s] -> RFPressureLow/1(task_time_s)
  [VPMM_PowerSta_enum] -> RFPressureLow/2(VPMM_PowerSta_enum)
  [DTC_clear_request] -> RFPressureLow/3(DTC_clear_request)
  [DTC_clear_request] -> LRPressureLow/3(DTC_clear_request)
  [VPMM_PowerSta_enum] -> LRPressureLow/2(VPMM_PowerSta_enum)
  [task_time_s] -> LRPressureLow/1(task_time_s)
  [task_time_s] -> RRPressureLow/1(task_time_s)
  [VPMM_PowerSta_enum] -> RRPressureLow/2(VPMM_PowerSta_enum)
  [DTC_clear_request] -> RRPressureLow/3(DTC_clear_request)
  LFPressureLow/1(VDDM_LFPressIndiDTC_raw32) -> VDDM_LFPressIndiDTC_raw32/1
  RFPressureLow/1(VDDM_RFPressIndiDTC_raw32) -> VDDM_RFPressIndiDTC_raw32/1
  LRPressureLow/1(VDDM_LRPressIndiDTC_raw32) -> VDDM_LRPressIndiDTC_raw32/1
  RRPressureLow/1(VDDM_RRPressIndiDTC_raw32) -> VDDM_RRPressIndiDTC_raw32/1
  VTPM_LFPressIndi_enum/1 -> LFPressureLow/4(VTPM_LFPressIndi_enum)
  VTPM_RFPressIndi_enum/1 -> RFPressureLow/4(VTPM_RFPressIndi_enum)
  VTPM_LRPressIndi_enum/1 -> LRPressureLow/4(VTPM_LRPressIndi_enum)
  VTPM_RRPressIndi_enum/1 -> RRPressureLow/4(VTPM_RRPressIndi_enum)
  [task_time_s] -> LFWheelTmpHigh/1(task_time_s)
  [VPMM_PowerSta_enum] -> LFWheelTmpHigh/2(VPMM_PowerSta_enum)
  [DTC_clear_request] -> LFWheelTmpHigh/3(DTC_clear_request)
  [task_time_s] -> RFWheelTmpHigh/1(task_time_s)
  [VPMM_PowerSta_enum] -> RFWheelTmpHigh/2(VPMM_PowerSta_enum)
  [DTC_clear_request] -> RFWheelTmpHigh/3(DTC_clear_request)
  [task_time_s] -> LRWheelTmpHigh/1(task_time_s)
  [VPMM_PowerSta_enum] -> LRWheelTmpHigh/2(VPMM_PowerSta_enum)
  [DTC_clear_request] -> LRWheelTmpHigh/3(DTC_clear_request)
  [task_time_s] -> RRWheelTmpHigh/1(task_time_s)
  [VPMM_PowerSta_enum] -> RRWheelTmpHigh/2(VPMM_PowerSta_enum)
  [DTC_clear_request] -> RRWheelTmpHigh/3(DTC_clear_request)
  VTPM_LFWheelTmpIndi_flg/1 -> LFWheelTmpHigh/4(VTPM_LFWheelTmpHigh_flg)
  VTPM_RFWheelTmpIndi_flg/1 -> RFWheelTmpHigh/4(VTPM_RFWheelTmpHigh_flg)
  VTPM_LRWheelTmpIndi_flg/1 -> LRWheelTmpHigh/4(VTPM_LRWheelTmpHigh_flg)
  VTPM_RRWheelTmpIndi_flg/1 -> RRWheelTmpHigh/4(VTPM_RRWheelTmpHigh_flg)
  LFWheelTmpHigh/1(VDDM_LFWheelTmpHighDTC_raw32) -> VDDM_LFWheelTmpHighDTC_raw32/1
  RFWheelTmpHigh/1(VDDM_RFWheelTmpHighDTC_raw32) -> VDDM_RFWheelTmpHighDTC_raw32/1
  LRWheelTmpHigh/1(VDDM_LRWheelTmpHighDTC_raw32) -> VDDM_LRWheelTmpHighDTC_raw32/1
  RRWheelTmpHigh/1(VDDM_RRWheelTmpHighDTC_raw32) -> VDDM_RRWheelTmpHighDTC_raw32/1
  [task_time_s] -> LFSensorfail/1(task_time_s)
  [VPMM_PowerSta_enum] -> LFSensorfail/2(VPMM_PowerSta_enum)
  [DTC_clear_request] -> LFSensorfail/3(DTC_clear_request)
  [task_time_s] -> RFSensorfail/1(task_time_s)
  [VPMM_PowerSta_enum] -> RFSensorfail/2(VPMM_PowerSta_enum)
  [DTC_clear_request] -> RFSensorfail/3(DTC_clear_request)
  [task_time_s] -> LRSensorfail/1(task_time_s)
  [VPMM_PowerSta_enum] -> LRSensorfail/2(VPMM_PowerSta_enum)
  [DTC_clear_request] -> LRSensorfail/3(DTC_clear_request)
  [task_time_s] -> RRSensorfail/1(task_time_s)
  [VPMM_PowerSta_enum] -> RRSensorfail/2(VPMM_PowerSta_enum)
  [DTC_clear_request] -> RRSensorfail/3(DTC_clear_request)
  VTPM_LFSensorFail_flg/1 -> LFSensorfail/4(VTPM_LFSensorFail_flg)
  VTPM_RFSensorFail_flg/1 -> RFSensorfail/4(VTPM_RFSensorFail_flg)
  VTPM_LRSensorFail_flg/1 -> LRSensorfail/4(VTPM_LRSensorFail_flg)
  VTPM_RRSensorFail_flg/1 -> RRSensorfail/4(VTPM_RRSensorFail_flg)
  LFSensorfail/1(VDDM_LFSensorFailDTC_raw32) -> VDDM_LFSensorFailDTC_raw32/1
  RFSensorfail/1(VDDM_RFSensorFailDTC_raw32) -> VDDM_RFSensorFailDTC_raw32/1
  LRSensorfail/1(VDDM_LRSensorFailDTC_raw32) -> VDDM_LRSensorFailDTC_raw32/1
  RRSensorfail/1(VDDM_RRSensorFailDTC_raw32) -> VDDM_RRSensorFailDTC_raw32/1
